simulink model "car_model_FIXED"  (R2022b)
settings: Solver=VariableStepAuto  StartTime=0.0  StopTime=60  RelTol=1e-3
values from neighbouring files (symbols this model uses):
  ABS_MAX_TORQUE = [25 25 25 25]    [Startup.m]
  ABS_MAX_TRQ_CMD = dot(ABS_MAX_TORQUE, MOTOR_ENABLE)    [Startup.m]
  ABS_MIN_TORQUE = [0.01 0.01 0.01 0.01]    [Startup.m]
  acc_IC = 0    [Startup.m]
  ACCELERATION_MAX = 30    [Startup.m]
  ang_IC = 0    [Startup.m]
  ang_vel_IC = 0    [Startup.m]
  ax = Reference_Signals.Chassis_Acceleration_VNED.ax.Data(:)    [Simulation_Data_Parse.m]    (also in Vehicle_Sim_Parse.m)
  ay = Reference_Signals.Chassis_Acceleration_VNED.ay.Data(:)    [Simulation_Data_Parse.m]    (also in Vehicle_Sim_Parse.m)
  az = Reference_Signals.Chassis_Acceleration_VNED.az.Data(:)    [Simulation_Data_Parse.m]    (also in Vehicle_Sim_Parse.m)
  battery_current_IC = 0    [Startup.m]
  BATTERY_CURRENT_MAX = 140    [Startup.m]
  BATTERY_CURRENT_MIN = 0    [Startup.m]
  battery_FT_IC = 300    [Startup.m]
  battery_T_IC = 300    [Startup.m]
  BATTERY_TEMPERATURE_MAX = 60    [Startup.m]
  BATTERY_TEMPERATURE_MIN = 0    [Startup.m]
  battery_voltage_IC = Ns*max(Em)    [Startup.m]
  BATTERY_VOLTAGE_MAX = 340    [Startup.m]
  BATTERY_VOLTAGE_MIN = 60    [Startup.m]
  Brake_Pressure_IC = 1    [Startup.m]
  ccl_IC = 0    [Startup.m]
  CENTER_STEER_ANGLE_MAX = 130    [Startup.m]
  covarience_matrix_IC = Simulink.Parameter(eye(28)./1000)    [Startup.m]
  dcl_IC = 140    [Startup.m]
  DCL_MAX = 130    [Startup.m]
  DCL_MIN = 0    [Startup.m]
  driver_t = 0.015    [Startup.m]
  fusion_t = Simulink.Parameter(0.01)    [Startup.m]
  fusion_t_sim = fusion_t.copy    [Startup.m]
  Fz_IC = m_all*g/4    [Startup.m]
  g = 9.81    [Startup.m]
  gps_hz = 0.01    [Startup.m]
  gps_ratio = Simulink.Parameter(gps_hz / imu_hz.Value)    [Startup.m]
  imu_hz = fusion_t.copy    [Startup.m]
  location_lla_IC = Simulink.Parameter([40.437675, -86.943750, 200])    [Startup.m]
  MAG_MAX = 200    [Startup.m]
  Max_Brake_Pressure = 10^8    (= 100000000)    [Startup.m]
  Max_Driver_Input = 1    [Startup.m]
  MAX_DTHETA_DRIVER = 360    [Startup.m]
  MAX_STEERING_ADJUST = 15    [Startup.m]
  Min_Brake_Pressure = 1    [Startup.m]
  Min_Driver_Input = 0    [Startup.m]
  motor_current_IC = 0    [Startup.m]
  MOTOR_CURRENT_MAX = 70    [Startup.m]
  MOTOR_CURRENT_MIN = 0    [Startup.m]
  MOTOR_ENABLE = [0 0 1 1]    [Startup.m]
  motor_FT_IC = 300    [Startup.m]
  motor_T_IC = 300    [Startup.m]
  MOTOR_TEMPERATURE_MAX = 100    [Startup.m]
  MOTOR_TEMPERATURE_MIN = 0    [Startup.m]
  motor_voltage_IC = 332    [Startup.m]
  MOTOR_VOLTAGE_MAX = 340    [Startup.m]
  MOTOR_VOLTAGE_MIN = 90    [Startup.m]
  omega_IC = 0    [Startup.m]
  OMEGA_MAX = 150    [Startup.m]
  OMEGA_MIN = 0    [Startup.m]
  ORIENTATION_MAX = 360    [Startup.m]
  pos_IC = 0    [Startup.m]
  POS_MAX = 300    [Startup.m]
  rho = 1.225    [Startup.m]
  selected_maxvm = MIN_TRACK_DATA.(event_names(10))    [Startup.m]
  selected_sweep = ALL_SWEEP_DATA.(sweep_names(1))    [Startup.m]
  selected_track = ALL_TRACK_DATA.(event_names(10))    [Startup.m]
  shock_length_IC = 0.1    [Startup.m]
  SHOCK_LENGTH_MAX = 0.25    [Startup.m]
  SHOCK_LENGTH_MIN = 0    [Startup.m]
  state_IC = zeros(28,1)    [Startup.m]
  theta_IC = 0    [Startup.m]
  TRACTION_ENABLE = 0    [Startup.m]
  TVS_ENABLE = 0    [Startup.m]
  tvs_t = 0.015    [Startup.m]
  tvs_t_sim = tvs_t    (= 0.015)    [Startup.m]
  Tx_I = 0    [Startup.m]
  vel_IC = [0 0 0]    [Startup.m]
  VELOCITY_MAX = 30    [Startup.m]
  X = Reference_Signals.Chassis_Position.X.Data(:)    [Simulation_Data_Parse.m]    (also in Vehicle_Sim_Parse.m = Chassis_Signals.InertFrm.Cg.Disp.X.Data(:))
  Y = Reference_Signals.Chassis_Position.Y.Data(:)    [Simulation_Data_Parse.m]    (also in Vehicle_Sim_Parse.m = Chassis_Signals.InertFrm.Cg.Disp.Y.Data(:))
  YAW_ENABLE = 1    [Startup.m]
  YAW_MAX = 2.5    [Startup.m]
undefined symbols (not defined in the file or in its folder): ActSuspDutyCycle, Aeq_left, Aeq_right, alpha_error, ang_acc_hystersesis, area_air, axb, br, brake_bias, covA, covG, covM, covP, covV, CURRENT_BUFFER, cy_sweep, dB, deadband_angle, dIndex, DiscIntNeverNeededParam, dt_OFF, dt_ON, dTx, dx, dZ, efficiency_grid, F0z, forward_look_straight, forward_look_turn, Fz_sweep, GAIN_ABS, gearbox_efficiency, gr, I, I_Driver, IMU_accel, IMU_gyro, IMU_mag, IMUNED2VNED, indicies, IYY, kx_sweep, l, lambda_star, low_V_SA, lr, m_all, m_body, m_unsprung, MAGNED2VNED, MAX_I_Driver, max_yaw, min_velocity_regen, motorControllerCurve, motorTempCurve, motorTempX, mu_star, mx_sweep, my_sweep, noise_state ... (+40)
libraries: fl_lib x82, nesl_utility x32, vehdynlibtire x10, vehdynlibsuspension x8, simulink x5, autolibutils x5, sharedtransform x5, sdl_lib x4, EngineCoolingComponents_lib x4, slpidlib x3, SimscapeFluids_lib x3, shared6dof x2
(part 14 of 14)

== system car_model_FIXED/Vehicle Model/Wheels and Tires/VDBS/Tires/MF Tires/Mx ==
  In1 : Inport
  In2 : Inport  Port=2
  In3 : Inport  Port=3
  In4 : Inport  Port=4
  Bus Selector{,1..3} (4 alike) : BusSelector  OutputSignals=Mx
  Vector Concatenate : Concatenate  NumInputs=4
  Out1 : Outport  VectorParamsAs1DForOutWhenUnconnected=off
  wires:
  Vector Concatenate/1 -> Out1/1
  In1/1 -> Bus Selector/1
  Bus Selector/1 -> Vector Concatenate/1  "<Mx>"
  In2/1 -> Bus Selector1/1
  In3/1 -> Bus Selector2/1
  In4/1 -> Bus Selector3/1
  Bus Selector1/1 -> Vector Concatenate/2  "<Mx>"
  Bus Selector2/1 -> Vector Concatenate/3  "<Mx>"
  Bus Selector3/1 -> Vector Concatenate/4  "<Mx>"

== system car_model_FIXED/Vehicle Model/Wheels and Tires/VDBS/Tires/MF Tires/My ==
  In1 : Inport
  In2 : Inport  Port=2
  In3 : Inport  Port=3
  In4 : Inport  Port=4
  Bus Selector{,1..3} (4 alike) : BusSelector  OutputSignals=My
  Vector Concatenate : Concatenate  NumInputs=4
  Out1 : Outport  VectorParamsAs1DForOutWhenUnconnected=off
  wires:
  Bus Selector3/1 -> Vector Concatenate/4  "<My>"
  Bus Selector2/1 -> Vector Concatenate/3  "<My>"
  Bus Selector1/1 -> Vector Concatenate/2  "<My>"
  In4/1 -> Bus Selector3/1
  In3/1 -> Bus Selector2/1
  In2/1 -> Bus Selector1/1
  Bus Selector/1 -> Vector Concatenate/1  "<My>"
  In1/1 -> Bus Selector/1
  Vector Concatenate/1 -> Out1/1

== system car_model_FIXED/Vehicle Model/Wheels and Tires/VDBS/Tires/MF Tires/Mz ==
  In1 : Inport
  In2 : Inport  Port=2
  In3 : Inport  Port=3
  In4 : Inport  Port=4
  Bus Selector{,1..3} (4 alike) : BusSelector  OutputSignals=Mz
  Vector Concatenate : Concatenate  NumInputs=4
  Out1 : Outport  VectorParamsAs1DForOutWhenUnconnected=off
  wires:
  Bus Selector3/1 -> Vector Concatenate/4  "<Mz>"
  Bus Selector2/1 -> Vector Concatenate/3  "<Mz>"
  Bus Selector1/1 -> Vector Concatenate/2  "<Mz>"
  In4/1 -> Bus Selector3/1
  In3/1 -> Bus Selector2/1
  In2/1 -> Bus Selector1/1
  Bus Selector/1 -> Vector Concatenate/1  "<Mz>"
  In1/1 -> Bus Selector/1
  Vector Concatenate/1 -> Out1/1

== system car_model_FIXED/Vehicle Model/Wheels and Tires/VDBS/Tires/MF Tires/Re ==
  In1 : Inport
  In2 : Inport  Port=2
  In3 : Inport  Port=3
  In4 : Inport  Port=4
  Bus Selector{,1..3} (4 alike) : BusSelector  OutputSignals=Re
  Vector Concatenate : Concatenate  NumInputs=4
  Out1 : Outport  VectorParamsAs1DForOutWhenUnconnected=off
  wires:
  Vector Concatenate/1 -> Out1/1
  In1/1 -> Bus Selector/1
  Bus Selector/1 -> Vector Concatenate/1  "<Re>"
  In2/1 -> Bus Selector1/1
  In3/1 -> Bus Selector2/1
  In4/1 -> Bus Selector3/1
  Bus Selector1/1 -> Vector Concatenate/2  "<Re>"
  Bus Selector2/1 -> Vector Concatenate/3  "<Re>"
  Bus Selector3/1 -> Vector Concatenate/4  "<Re>"

== system car_model_FIXED/Vehicle Model/Wheels and Tires/VDBS/Tires/MF Tires/alpha ==
  In1 : Inport
  In2 : Inport  Port=2
  In3 : Inport  Port=3
  In4 : Inport  Port=4
  Bus Selector{,1..3} (4 alike) : BusSelector  OutputSignals=Alpha
  Vector Concatenate : Concatenate  NumInputs=4
  Out1 : Outport  VectorParamsAs1DForOutWhenUnconnected=off
  wires:
  Vector Concatenate/1 -> Out1/1
  In1/1 -> Bus Selector/1
  Bus Selector/1 -> Vector Concatenate/1  "<Alpha>"
  In2/1 -> Bus Selector1/1
  In3/1 -> Bus Selector2/1
  In4/1 -> Bus Selector3/1
  Bus Selector1/1 -> Vector Concatenate/2  "<Alpha>"
  Bus Selector2/1 -> Vector Concatenate/3  "<Alpha>"
  Bus Selector3/1 -> Vector Concatenate/4  "<Alpha>"

== system car_model_FIXED/Vehicle Model/Wheels and Tires/VDBS/Tires/MF Tires/kappa ==
  In1 : Inport
  In2 : Inport  Port=2
  In3 : Inport  Port=3
  In4 : Inport  Port=4
  Bus Selector{,1..3} (4 alike) : BusSelector  OutputSignals=Kappa
  Vector Concatenate : Concatenate  NumInputs=4
  Out1 : Outport  VectorParamsAs1DForOutWhenUnconnected=off
  wires:
  Bus Selector3/1 -> Vector Concatenate/4  "<Kappa>"
  Bus Selector2/1 -> Vector Concatenate/3  "<Kappa>"
  Bus Selector1/1 -> Vector Concatenate/2  "<Kappa>"
  In4/1 -> Bus Selector3/1
  In3/1 -> Bus Selector2/1
  In2/1 -> Bus Selector1/1
  Bus Selector/1 -> Vector Concatenate/1  "<Kappa>"
  In1/1 -> Bus Selector/1
  Vector Concatenate/1 -> Out1/1

== system car_model_FIXED/Vehicle Model/Wheels and Tires/VDBS/Tires/MF Tires/omega ==
  In1 : Inport
  In2 : Inport  Port=2
  In3 : Inport  Port=3
  In4 : Inport  Port=4
  Bus Selector{,1..3} (4 alike) : BusSelector  OutputSignals=Omega
  Vector Concatenate : Concatenate  NumInputs=4
  Out1 : Outport  VectorParamsAs1DForOutWhenUnconnected=off
  wires:
  In1/1 -> Bus Selector/1
  Bus Selector/1 -> Vector Concatenate/1  "<Omega>"
  In2/1 -> Bus Selector1/1
  In3/1 -> Bus Selector2/1
  In4/1 -> Bus Selector3/1
  Bus Selector1/1 -> Vector Concatenate/2  "<Omega>"
  Bus Selector2/1 -> Vector Concatenate/3  "<Omega>"
  Bus Selector3/1 -> Vector Concatenate/4  "<Omega>"
  Vector Concatenate/1 -> Out1/1

== system car_model_FIXED/Vehicle Model/Wheels and Tires/VDBS/Tires/MF Tires/z ==
  In1 : Inport
  In2 : Inport  Port=2
  In3 : Inport  Port=3
  In4 : Inport  Port=4
  Bus Selector{,1..3} (4 alike) : BusSelector  OutputSignals=z
  Vector Concatenate : Concatenate  NumInputs=4
  Out1 : Outport  VectorParamsAs1DForOutWhenUnconnected=off
  wires:
  Bus Selector3/1 -> Vector Concatenate/4  "<z>"
  Bus Selector2/1 -> Vector Concatenate/3  "<z>"
  Bus Selector1/1 -> Vector Concatenate/2  "<z>"
  In4/1 -> Bus Selector3/1
  In3/1 -> Bus Selector2/1
  In2/1 -> Bus Selector1/1
  Bus Selector/1 -> Vector Concatenate/1  "<z>"
  In1/1 -> Bus Selector/1
  Vector Concatenate/1 -> Out1/1

== system car_model_FIXED/Vehicle Model/Wheels and Tires/VDBS/Tires/MF Tires/zdot ==
  In1 : Inport
  In2 : Inport  Port=2
  In3 : Inport  Port=3
  In4 : Inport  Port=4
  Bus Selector{,1..3} (4 alike) : BusSelector  OutputSignals=zdot
  Vector Concatenate : Concatenate  NumInputs=4
  Out1 : Outport  VectorParamsAs1DForOutWhenUnconnected=off
  wires:
  Vector Concatenate/1 -> Out1/1
  In1/1 -> Bus Selector/1
  Bus Selector/1 -> Vector Concatenate/1  "<zdot>"
  In2/1 -> Bus Selector1/1
  In3/1 -> Bus Selector2/1
  In4/1 -> Bus Selector3/1
  Bus Selector1/1 -> Vector Concatenate/2  "<zdot>"
  Bus Selector2/1 -> Vector Concatenate/3  "<zdot>"
  Bus Selector3/1 -> Vector Concatenate/4  "<zdot>"

== matlab function car_model_FIXED/Vehicle Model/Vehicle/6DOF/Suspension to Chasiss Transforms/Estimated Unsprung Mass Orientation ==
  data: angles output size=3; angleIn input size=3; GeomXYZ output size=3; GemoXYZIn input size=3; Ground input size=4; trackW parameter; wheelB parameter
function [angles,GeomXYZ]= three26(angleIn, GemoXYZIn, Ground,trackW, wheelB)%#codegen
coder.allowpcode('plain')
% Copyright 2018 The MathWorks, Inc.
[angles,GeomXYZ]= vdynthree2six(angleIn, GemoXYZIn, Ground,trackW, wheelB);

== matlab function car_model_FIXED/Driver & Environment/Reference Generator/Reference Geneator ==
  data: index_small input; index_all input; psi input; deg2rad parameter; Vg input; yaw input; pos input; omega input; index_small output; index_all output; v_error output; d_error output; psi_error output; v_cog output; r_ref output; r_error output; x_ref output; y_ref output; yaw_ref output; omega output; p_error output; Vnow output; ahead output; ahead input; selected_track parameter; dIndex parameter; dx parameter; forward_look_straight parameter; forward_look_turn parameter; q_thresh parameter; indicies parameter; selected_maxvm parameter; axb parameter; di_now output; di_prev input
function [index_small, index_all, v_error, d_error, psi_error, v_cog, r_ref, r_error, x_ref, y_ref, yaw_ref, omega, p_error,Vnow, ahead, di_now] = ref_gen(index_small, index_all, psi, deg2rad, Vg, yaw, pos, omega, ahead, selected_track, dIndex, dx, forward_look_straight, forward_look_turn, q_thresh, indicies, selected_maxvm, axb, di_prev)
%% Extract Data
Y_all = selected_track(index_all:index_all+dIndex,2);
X_all = selected_track(index_all:index_all+dIndex,3);

Vmax_now = selected_maxvm(index_small,3);
num_elem = length(selected_maxvm(:,1));

if num_elem > index_small
    Vmax_next = selected_maxvm(index_small+1,3);
    d_next = selected_maxvm(index_small+1,1);
else
    Vmax_next = Vmax_now;
    d_next = 100;
end

%% Determine Reference Point
d_error_all = sqrt((Y_all - pos.Y).^2 + (X_all - pos.X).^2);
[min_d, min_index] = min(d_error_all);
index_all = index_all + min_index - 1;

%% Aquire Reference Values
y_ref = selected_track(index_all, 2);
x_ref = selected_track(index_all, 3);
y_ref_next = selected_track(index_all+5, 2);
x_ref_next = selected_track(index_all+5, 3);
r_ref = selected_track(index_all, 4);
r_straight = selected_track(index_all+forward_look_straight, 4);
r_turn = selected_track(index_all+forward_look_turn, 4);
turn_ref = selected_track(index_all, 5);
straight_next = selected_track(index_all+forward_look_straight, 5);
turn_next = selected_track(index_all+forward_look_turn, 5);
psi_ref = selected_track(index_all, 8);
di_now = selected_track(index_all, 9);

%% Velocity Error
v_cog = sqrt((Vg.xdot^2) + (Vg.ydot^2));

if ahead
    di = (di_now*dx) + d_next;
else
    di = di_now*dx;
end

det = v_cog^2 + (2*axb*di);

if det < 0
    Vnext = 0;
else
    Vnext = sqrt(det);
end

increment = 0;

if (abs(Vmax_next - Vnext) < 0.25) && (Vmax_now > Vmax_next) && (~ahead)
    Vnow = Vmax_next;
    index_small = index_small + 1;
    ahead = 1;
    increment = 1;
elseif ((di_now - di_prev) > 0) && ~ahead
    Vnow = Vmax_next;
    index_small = index_small + 1;
else
    Vnow = Vmax_now;
end

if ((di_now - di_prev) > 0) && ~increment
    ahead = 0;
end

% if r_ref ~= inf
%     Vnow = min(Vnow, 17);
% end

v_error = Vnow - v_cog - 1;

%% Turning Radius Error
if (turn_ref ~= straight_next) || (r_ref ~= r_straight)
    turn_ref = straight_next;
    r_ref = r_straight;
elseif (turn_ref ~= turn_next) && (turn_next ~= 0) && (turn_ref ~= 0)
    turn_ref = turn_next;
    r_ref = r_turn;
end

r_IC = abs(v_cog / yaw);
r_error = turn_ref *  ((1 / r_ref) - (1 / r_IC));

if r_ref == inf
    yaw_ref = 0;
else
    yaw_ref = turn_ref * v_cog / r_ref;
end

%% Angle Error
sign_steer = 1;

if (abs(psi - psi_ref) > pi) && (sign(psi) ~= sign(psi_ref))
    if psi < 0
        sign_steer = -1;
    end
elseif (psi > psi_ref)
    sign_steer = -1;   
end

if abs(psi_ref - psi) < pi
    psi_error = sign_steer * abs(psi_ref - psi) / deg2rad;
else
    psi_error = sign_steer * ((pi - abs(psi_ref)) + (pi - abs(psi))) / deg2rad;
end

%% Distance Error
% Determine Vehicle Quadrant
if (pos.Y - y_ref) > q_thresh
   if (pos.X - x_ref) > q_thresh
       Qc = 5;
   elseif (pos.X - x_ref) < -q_thresh
       Qc = 11;
   else
       Qc = 4;
   end
elseif (pos.Y - y_ref) < -q_thresh
   if (pos.X - x_ref) > q_thresh
       Qc = 7;
   elseif (pos.X - x_ref) < -q_thresh
       Qc = 9;
   else
       Qc = 8;
   end
else
   if (pos.X - x_ref) > q_thresh
       Qc = 6;
   elseif (pos.X - x_ref) < -q_thresh
       Qc = 10;
   else
       Qc = 0;
   end
end

% Determine Next Reference Point Quadrant
if y_ref_next > y_ref
   if x_ref_next > x_ref
       Qn = 5;
   elseif x_ref_next < x_ref
       Qn = 11;
   else
       Qn = 4;
   end
elseif y_ref_next < y_ref
   if x_ref_next > x_ref
       Qn = 7;
   elseif x_ref_next < x_ref
       Qn = 9;
   else
       Qn = 8;
   end
else
   if x_ref_next > x_ref
       Qn = 6;
   elseif x_ref_next < x_ref
       Qn = 10;
   else
       Qn = 0;
   end
end

% Determine Sign for Distance Error
if Qc == 0
   sign_distance = 0;
elseif (abs(x_ref_next - x_ref) == abs(pos.X - x_ref)) && (abs(y_ref_next - y_ref) == abs(pos.Y - y_ref))
   sign_distance = 0;
elseif ((Qc ~= Qn) && (indicies(Qc+4) ~= Qn))
    if (indicies(Qc+1) == indicies(Qn)) || (indicies(Qc+2) == indicies(Qn)) || (indicies(Qc+3) == indicies(Qn))
        sign_distance = -1;
    else
        sign_distance = 1;
    end
else
    if indicies(Qc) == 1 || indicies(Qc) == 3
        y_axis = y_ref;
    elseif indicies(Qc) == 4
        y_axis = y_ref + 1;
    else
        y_axis = y_ref - 1;
    end
    
    if indicies(Qc) == 2 || indicies(Qc) == 4
        x_axis = x_ref;
    elseif indicies(Qc) == 1
        x_axis = x_ref + 1;
    else
        x_axis = x_ref - 1;
    end
    
    axis_coordiantes = [y_axis, x_axis];
    ref_coordiantes = [y_ref, x_ref];
    next_ref_coordinates = [y_ref_next, x_ref_next];
    vehicle_coordinates = [pos.Y, pos.X];
    
    ref_vec = axis_coordiantes - ref_coordiantes;
    veh_vec = vehicle_coordinates - ref_coordiantes;
    next_ref = next_ref_coordinates - ref_coordiantes;
    
    theta_veh_ref = acos(dot(ref_vec, veh_vec) / (norm(ref_vec)*norm(veh_vec)));
    theta_next_ref = acos(dot(ref_vec, next_ref) / (norm(ref_vec)*norm(next_ref)));
    
    if theta_veh_ref < theta_next_ref
        sign_distance = 1;
    else
        sign_distance = -1;
    end
end

d_error = sign_distance * min_d;

%% Combined Purtubation Error
if (sign_distance~=sign(psi_error)) && (d_error~=0)
    p_error = d_error;
else
    p_error = psi_error;
end

end

== matlab function car_model_FIXED/Driver & Environment/Longitudinal Control/ABS/ABS system/MATLAB Function1 ==
  data: u input; y output; mu_star parameter; lambda_star parameter
function y = fcn(u,mu_star, lambda_star)

    y = (2.*mu_star.*lambda_star.*u./(lambda_star.^2+u.^2));

end

== matlab function car_model_FIXED/Driver & Environment/Sweep Generator/Sweep Generator ==
  data: index input; index output; vel input; ON input; vel_err output; ref_steer output; ON output; selected_sweep parameter; dt_ON parameter; dt_OFF parameter; counter output; counter input; tvs_t_sim parameter
function [index, vel_err,ref_steer, ON, counter] = fcn(index, vel, ON, selected_sweep, dt_ON, dt_OFF, counter, tvs_t_sim)

% Update Control Output
ref_vel = selected_sweep(index, 1);
ref_steer = selected_sweep(index, 2);
vel_err = ref_vel - norm([vel.xdot vel.ydot]);
counter = counter + 1;

% Update Scenario
if ((counter*tvs_t_sim) == dt_ON && ON) || ((counter*tvs_t_sim) == dt_OFF && ~ON)
    index = index + 1;
    counter = 0;

    if (selected_sweep(index, 2) == 0 && index > 1)
        ON = double(~ON);
    end

end

== matlab function car_model_FIXED/Vehicle Model/Vehicle/6DOF/Suspension to Chasiss Transforms/MATLAB Function ==
  data: u input; y output; aero_coeff parameter
function y = fcn(u, aero_coeff)

Fz = aero_coeff*u^2;


y = [0 0 Fz];

== matlab function car_model_FIXED/Vehicle Model/Electronics/Navigation Sensors/VNED to SNED ==
  data: accel_SNED output; gyro_SNED output; accel_VNED input size=[3 1]; gyro_VNED input size=[3 1]; mag_VNED input size=[3 1]; mag_SNED output; phi parameter
function [accel_SNED, gyro_SNED, mag_SNED] = VNED2SNED(accel_VNED, gyro_VNED, mag_VNED, phi)
%% Define Rotation
IMUNED2VNED = rotmat(quaternion([0 (phi - 180) 0],"eulerd","XYZ","frame"),"frame");
MAGNED2VNED = rotmat(quaternion([180 (180 - phi) 0],"eulerd","XYZ","frame"),"frame");

%% Coordinate Transformation
accel_SNED = IMUNED2VNED\accel_VNED;
gyro_SNED = IMUNED2VNED\gyro_VNED;
mag_SNED = MAGNED2VNED\mag_VNED;

end

== matlab function car_model_FIXED/Vehicle Model/Electronics/Navigation Sensors/integrate angvel ==
  data: Orientation_e input; Orientation_c output; Orientation_e output
function [Orientation_c, Orientation_e]  = fcn(Orientation_e)

Orientation_q = quaternion(Orientation_e, 'euler', 'XYZ', 'frame');

Orientation_c = compact(Orientation_q);

end

== matlab function car_model_FIXED/Control Systems/Sensor Fusion/SFS/fusion ==
  data: state_out output; state_in input; rot_map output [-4..4]; ang output; angvel output; pos output; vel output; accel output; mag output; accel_bias output; gyro_bias output; mag_bias output; velocity input size=[3 1] [-VELOCITY_MAX..VELOCITY_MAX]; position input size=[3 1] [-POS_MAX..POS_MAX]; acceleration input size=[3 1] [-ACCELERATION_MAX..ACCELERATION_MAX]; angularVelocity input size=[3 1] [-YAW_MAX..YAW_MAX]; magField input size=[3 1] [-MAG_MAX..MAG_MAX]; cov_in input [-10..10]; covG parameter; covA parameter; covM parameter; covP parameter; covV parameter; fusion_t parameter; location_lla_IC parameter; cov_out output [-10..10]; noise_state parameter; gps_ratio parameter
function [state_out, rot_map, ang, angvel, pos, vel, accel, mag, accel_bias, gyro_bias, mag_bias, cov_out] = fusion(state_in, velocity, position ,acceleration,angularVelocity, magField, cov_in, covG, covA, covM, covP, covV, fusion_t, location_lla_IC, noise_state, gps_ratio) 
%% Create Filter
filter = insfilterAsync();
filter.ReferenceLocation = location_lla_IC;
filter.State = state_in;
filter.StateCovariance = cov_in;

filter.QuaternionNoise = noise_state(1:4);
filter.AngularVelocityNoise = noise_state(5:7);
filter.PositionNoise = noise_state(8:10);
filter.VelocityNoise = noise_state(11:13);
filter.AccelerationNoise = noise_state(14:16);
filter.GyroscopeBiasNoise = noise_state(17:19);
filter.AccelerometerBiasNoise = noise_state(20:22);
filter.GeomagneticVectorNoise = noise_state(23:25);
filter.MagnetometerBiasNoise = noise_state(26:28);

%% Sensor Fusion
predict(filter, fusion_t);

fuseaccel(filter,acceleration',covA);
fusegyro(filter,angularVelocity',covG);
fusemag(filter, magField',covM);
fusegps(filter,position',covP,velocity',covV);

[~,rot_map,~] = pose(filter, 'rotmat');

%% Save Fusion State & State Covariance
state_out = filter.State;
cov_out = filter.StateCovariance;

%% Extract Individual Signals
% Vehicle POSE
ang = state_out(1:4);                    % quaternion (VNED2SNED)
angvel = state_out(5:7);                 % chassis angular velocity (rad/s)(VNED)
pos = state_out(8:10);                   % chassis position (m)(NED)
vel = state_out(11:13);                  % chassis velocity (m/s)(VNED)
accel = state_out(14:16);                % chassis acceleration (m/s^2)(VNED)
mag = state_out(23:25);                  % magnetic field (uT)(NED)

% Sensor Parameters
accel_bias = state_out(17:19);           % accelerometer bias (m/s^2)(VNED)
gyro_bias = state_out(20:22);            % gyroscope bias (rad/s)(VNED)
mag_bias = state_out(26:28);             % magnetometer bias (uT)(NED)

end

== matlab function car_model_FIXED/Driver & Environment/Longitudinal Control/ABS/ABS system/MATLAB Function ==
  data: w_fake input; w input size=[1 4]; v input; tau output; lambda0 input size=[1 4]; vdot input; lambda input size=[1 4]; m_all parameter; RE parameter; IYY parameter; br parameter; d output
function [tau, d]  = fcn(w_fake,w,v,lambda0,vdot,lambda,m_all,RE,IYY,br)

if v > 0
    t1 = -IYY*v./RE.*(lambda-lambda0);
    t2 = -IYY.*w_fake./v.*vdot;
    t3 = -br.*w_fake;
    t4 = -(m_all.*RE.*vdot/4);
    tau = -IYY*v./RE.*(lambda-lambda0)-br.*w_fake-IYY.*w_fake./v.*vdot-(m_all.*RE.*vdot/4);
else
    tau = [0 0 0 0];
    t1 = [0 0 0 0];
    t2 = [0 0 0 0];
    t3 = [0 0 0 0];
    t4 = 0;
end

d1 = sqrt(abs((w(1)^2 - w(3)^2)/w(1)^2));
d2 = sqrt(abs((w(2)^2 - w(4)^2)/w(2)^2));

d = (min(max(d1, d2), 1));

if (w(3) < 3)
    d = 1;
elseif d > 0.5
    d = 0.5;
else
    d = 1;
end
